simulink model "robot_control_model"  (R2018b)
settings: Solver=FixedStepAuto  StartTime=0.0  StopTime=t_sim  FixedStep=dt  RelTol=1e-3
values from neighbouring files (symbols this model uses):
  F_amp = 0.1    [robot_control.m]
  f_F = 2    [robot_control.m]
  g = 9.81    [robot_control.m]
  G_s_denom = [-J/(m*g*l) 0 1]    [robot_control.m]
  G_s_num = [1/(m*g)]    [robot_control.m]
  J = m*l^2    (= 0.04)    [robot_control.m]
  KD = 3    [robot_control.m]
  KI = 0    [robot_control.m]
  KP = -50    [robot_control.m]
  l = 0.2    [robot_control.m]
  m = 1    [robot_control.m]
  phi_start = 0    [robot_control.m]
  w_start = 0    [robot_control.m]
settings Model: Creator=pgehr  LastModifiedBy=pgehr

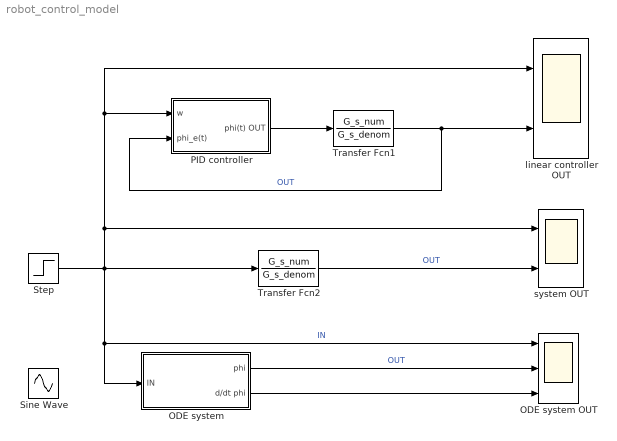
== system robot_control_model ==
  ODE system : Subsystem
  ODE system OUT : Scope  NumInputPorts=3
  PID controller : Subsystem
  Sine Wave : Sin  Amplitude=F_amp  Frequency=2*pi*f_F  SampleTime=0
  Step : Step  SampleTime=0
  Transfer Fcn1 : TransferFcn  Numerator=G_s_num  Denominator=G_s_denom
  Transfer Fcn2 : TransferFcn  Numerator=G_s_num  Denominator=G_s_denom
  linear controller OUT : Scope  NumInputPorts=2
  system OUT : Scope  NumInputPorts=2
  wires:
  Transfer Fcn1/1 -> PID controller/2(phi_e(t)), linear controller OUT/2  "OUT"
  PID controller/1(phi(t) OUT) -> Transfer Fcn1/1
  ODE system/1(phi) -> ODE system OUT/2  "OUT"
  Step/1 -> Transfer Fcn2/1, ODE system/1(IN), ODE system OUT/1, linear controller OUT/1, PID controller/1(w), system OUT/1  "IN"
  ODE system/2(d/dt phi) -> ODE system OUT/3
  Transfer Fcn2/1 -> system OUT/2  "OUT"

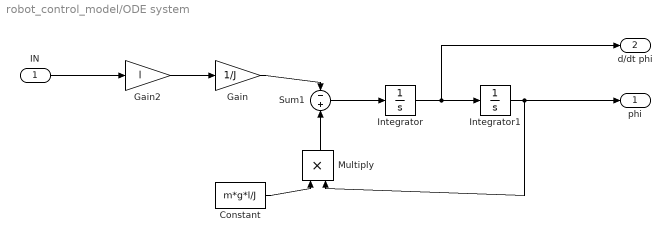
== system robot_control_model/ODE system ==
  IN : Inport
  Constant : Constant  Value=m*g*l/J
  Gain : Gain  Gain=1/J
  Gain2 : Gain  Gain=l
  Integrator : Integrator  InitialCondition=w_start
  Integrator1 : Integrator  InitialCondition=phi_start
  Multiply : Product  Inputs=**
  Sum1 : Sum  Inputs=-+
  phi : Outport
  d/dt phi : Outport  Port=2
  wires:
  Sum1/1 -> Integrator/1
  Integrator/1 -> d/dt phi/1, Integrator1/1
  Multiply/1 -> Sum1/2
  Gain/1 -> Sum1/1
  Constant/1 -> Multiply/1
  Integrator1/1 -> phi/1, Multiply/2
  IN/1 -> Gain2/1
  Gain2/1 -> Gain/1

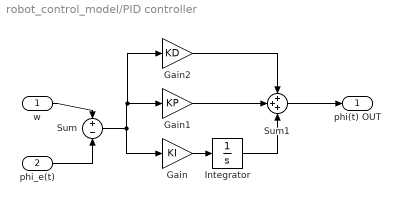
== system robot_control_model/PID controller ==
  w : Inport
  phi_e(t) : Inport  Port=2
  Gain : Gain  Gain=KI
  Gain1 : Gain  Gain=KP
  Gain2 : Gain  Gain=KD
  Integrator : Integrator
  Sum : Sum  Inputs=+-
  Sum1 : Sum  Inputs=+++
  phi(t) OUT : Outport
  wires:
  w/1 -> Sum/1
  phi_e(t)/1 -> Sum/2
  Sum1/1 -> phi(t) OUT/1
  Gain/1 -> Integrator/1
  Sum/1 -> Gain/1, Gain2/1, Gain1/1
  Gain2/1 -> Sum1/1
  Integrator/1 -> Sum1/3
  Gain1/1 -> Sum1/2
